simulink model "kontr_toka"  (R2023b)
settings: Solver=VariableStepAuto  StartTime=0.0  StopTime=0.01  MaxStep=0.000001  RelTol=1e-3
settings Model: Creator=volko  LastModifiedBy=volko

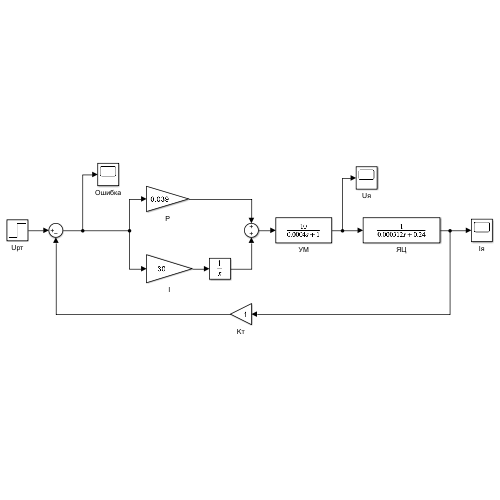
[thumbnail: Simulink's stored preview of the top-level diagram]
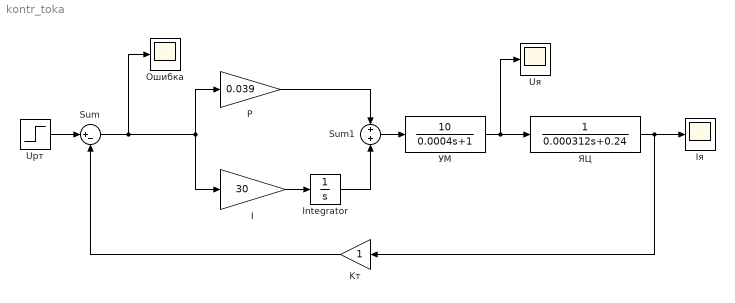
== system kontr_toka ==
  I : Gain  Gain=30
  Integrator : Integrator
  Iя : Scope
  Kт : Gain
  P : Gain  Gain=0.039
  Sum : Sum  Inputs=|+-
  Sum1 : Sum
  Uрт : Step  Time=0  SampleTime=0
  Uя : Scope
  Ошибка : Scope
  УМ : TransferFcn  Numerator=[10]  Denominator=[0.0004 1]
  ЯЦ : TransferFcn  Denominator=[0.000312 0.24]
  wires:
  Uрт/1 -> Sum/1
  УМ/1 -> Uя/1, ЯЦ/1
  Integrator/1 -> Sum1/2
  ЯЦ/1 -> Iя/1, Kт/1
  Kт/1 -> Sum/2
  Sum1/1 -> УМ/1
  I/1 -> Integrator/1
  Sum/1 -> Ошибка/1, I/1, P/1
  P/1 -> Sum1/1
